simulink model "Translation_X_Y_Sim"  (Simulink 7.5)
settings: Solver=ode45  StartTime=0.0  StopTime=10.0  RelTol=1e-3
undefined symbols (not defined in the file or in its folder): m
settings Model: Creator=roczit00  LastModifiedBy=Dio
settings DebuggingCC: StrictBusMsg=Warning

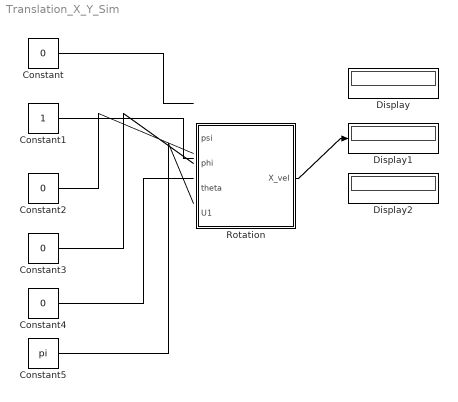
== system Translation_X_Y_Sim ==
  Constant{,2..4} (4 alike) : Constant  Value=0  OutDataType=fixdt(1, 16)  OutScaling=2^0
  Constant1 : Constant  OutDataType=fixdt(1, 16)  OutScaling=2^0
  Constant5 : Constant  Value=pi  OutDataType=fixdt(1, 16)  OutScaling=2^0
  Display : Display
  Display1 : Display
  Display2 : Display
  Rotation : Subsystem
  wires:
  Constant/1 -> ?
  Constant1/1 -> ?
  Constant2/1 -> ?
  ? -> Display/1
  Rotation/1(X_vel) -> Display1/1
  ? -> Display2/1
  Constant3/1 -> ?
  Constant4/1 -> ?
  Constant5/1 -> ?

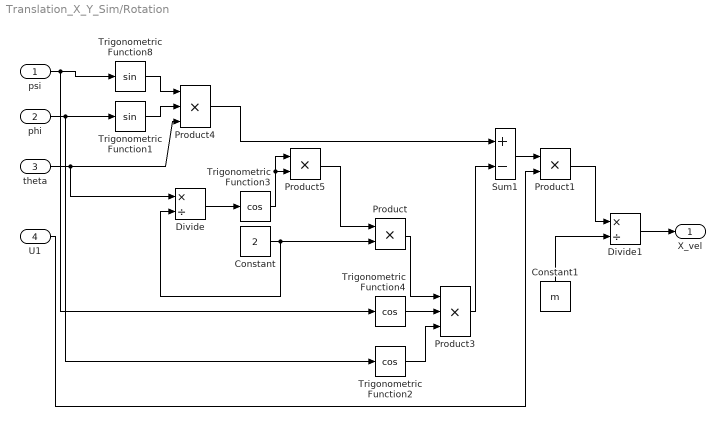
== system Translation_X_Y_Sim/Rotation ==
  psi : Inport  OutDataType=fixdt(1, 16)  OutScaling=2^0
  phi : Inport  Port=2  OutDataType=fixdt(1, 16)  OutScaling=2^0
  theta : Inport  Port=3  OutDataType=fixdt(1, 16)  OutScaling=2^0
  U1 : Inport  Port=4  OutDataType=fixdt(1, 16)  OutScaling=2^0
  Constant : Constant  Value=2  OutDataType=fixdt(1, 16)  OutScaling=2^0
  Constant1 : Constant  Value=m
  Divide : Product  Inputs=*/  OutDataType=fixdt(1, 16)  OutScaling=2^-10
  Divide1 : Product  Inputs=*/  OutDataType=fixdt(1, 16)  OutScaling=2^-10
  Product : Product  OutDataType=fixdt(1, 16)  OutScaling=2^0  RndMeth=Zero
  Product1 : Product  OutDataType=fixdt(1, 16)  OutScaling=2^0  RndMeth=Zero
  Product3 : Product  Inputs=3  OutDataType=fixdt(1, 16)  OutScaling=2^0  RndMeth=Zero
  Product4 : Product  Inputs=3  OutDataType=fixdt(1, 16)  OutScaling=2^0  RndMeth=Zero
  Product5 : Product  OutDataType=fixdt(1, 16)  OutScaling=2^0  RndMeth=Zero
  Sum1 : Sum  Inputs=+-  OutDataType=fixdt(1, 16)  OutScaling=2^0
  Trigonometric Function1 : Trigonometry
  Trigonometric Function2 : Trigonometry  Operator=cos
  Trigonometric Function3 : Trigonometry  Operator=cos
  Trigonometric Function4 : Trigonometry  Operator=cos
  Trigonometric Function8 : Trigonometry
  X_vel : Outport  OutDataType=fixdt(1, 16)  OutScaling=2^0
  wires:
  Trigonometric Function4/1 -> Product3/2
  Trigonometric Function2/1 -> Product3/3
  Trigonometric Function8/1 -> Product4/1
  Trigonometric Function1/1 -> Product4/2
  Product4/1 -> Sum1/1
  Product3/1 -> Sum1/2
  phi/1 -> Trigonometric Function1/1, Trigonometric Function2/1
  psi/1 -> Trigonometric Function8/1, Trigonometric Function4/1
  theta/1 -> Product4/3, Divide/1
  Constant/1 -> Product/2, Divide/2
  Product/1 -> Product3/1
  Divide/1 -> Trigonometric Function3/1
  Trigonometric Function3/1 -> Product5/1, Product5/2
  Product5/1 -> Product/1
  Sum1/1 -> Product1/1
  U1/1 -> Product1/2
  Product1/1 -> Divide1/1
  Constant1/1 -> Divide1/2
  Divide1/1 -> X_vel/1
